simulink model "tutorial_picooz_simulation"  (R2024a)
settings: Solver=ode45  StartTime=0.0  StopTime=22  MaxStep=.002  RelTol=1e-3  EnableMultiTasking=on
undefined symbols (not defined in the file): DiscIntNeverNeededParam
libraries: simulink x2
settings Model: Creator=M91449  LastModifiedBy=Lubin Kerhuel
settings SolverCC: AlgebraicLoopSolver=TrustRegion
settings DataIOCC: ExternalInput=getinputstruct(op_trim1)  InitialState=getstatestruct(op_trim1)  SaveFormat=Array  SaveOutput=off  DSMLogging=off  SaveTime=off  ReturnWorkspaceOutputs=off
settings OptimizationCC: LifeSpan=inf
settings DebuggingCC: UnderspecifiedInitializationDetection=Classic  MergeDetectMultiDrivingBlocksExec=none  SolverPrmCheckMsg=warning  UnconnectedInputMsg=warning  UnconnectedOutputMsg=warning  UnconnectedLineMsg=warning  StateNameClashWarn=warning  SFUnexpectedBacktrackingDiag=warning  SFNoUnconditionalDefaultTransitionDiag=warning  SFExecutionAtInitializationDiag=none  ArithmeticOperatorsInVariantConditions=warning
settings HardwareCC: ProdBitPerPointer=32  ProdBitPerSizeT=32  ProdBitPerPtrDiffT=32  ProdLargestAtomicFloat=None  ProdIntDivRoundTo=Undefined  ProdEndianess=Unspecified  ProdWordSize=32  ProdHWDeviceType=32-bit Generic
settings ModelReferenceCC: PropagateSignalLabelsOutOfModel=off
settings SFSimCC: SimUseLocalCustomCode=off  CustomCodeUndefinedFunction=UseInterfaceOnly
settings RTWCC: RTWUseLocalCustomCode=off  GPUComputeCapability=3.5
settings CodeAppCC: StateflowObjectComments=on
settings GRTTargetCC: TargetLangStandard=C89/C90 (ANSI)
settings ConfigComp: CovMetricSettings=dw  CovSaveCumulativeToWorkspaceVar=on  CovSaveSingleToWorkspaceVar=on  CovExternalEMLEnable=off  CovSFcnEnable=off

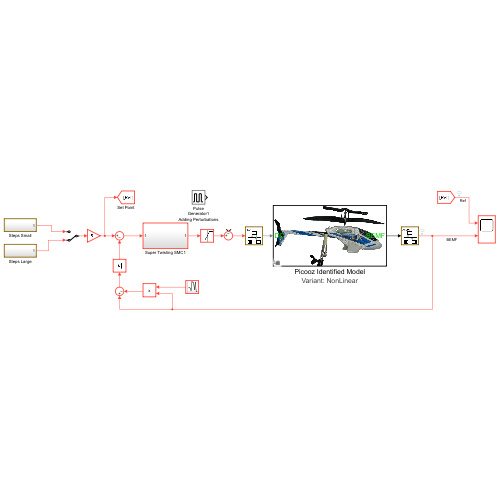
[thumbnail: Simulink's stored preview of the top-level diagram]
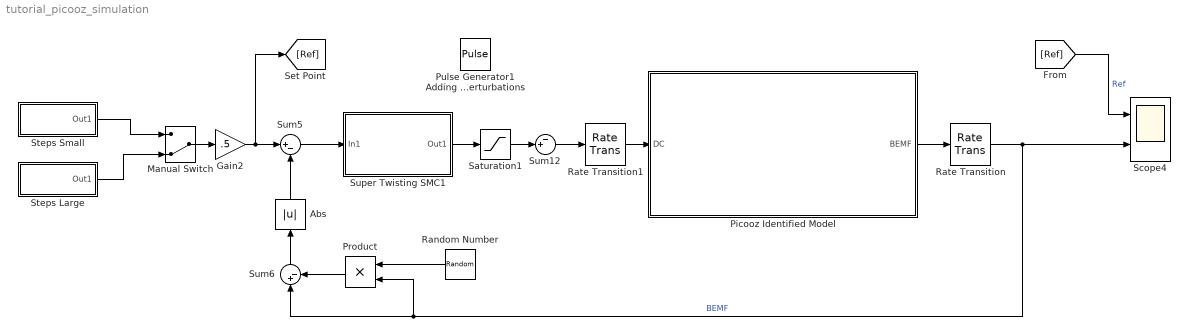
== system tutorial_picooz_simulation ==
  Abs : Abs  SaturateOnIntegerOverflow=off
  Gain2 : Gain  Gain=.5  OutDataTypeStr=double
  Manual Switch : ManualSwitch  CurrentSetting=0
  Picooz Identified Model : Subsystem  Variant=on  VariantControlMode=label  LabelModeActiveChoice=NonLinear
      settings: AttributesFormatString=Variant: %<ActiveVariant>
      mask Display:
      | color('green');
      | image('Picooz_01_Close.jpg');
      | port_label('input',1,'DC');
      | port_label('output',1,'BEMF');
      | %disp(get_param(gcb,'ActiveVariant'));
  Product : Product
  Pulse Generator1 Adding Perturbations : DiscretePulseGenerator  PulseType=Time based  Amplitude=.15  Period=2.3  PulseWidth=10
  Random Number : RandomNumber  Variance=.012^2*5  SampleTime=0.001
  Rate Transition : RateTransition  OutPortSampleTime=.001
  Rate Transition1 : RateTransition  OutPortSampleTime=0
  Saturation1 : Saturate  UpperLimit=.8  LowerLimit=0
  Scope4 : Scope  NumInputPorts=2
  Steps Large : Subsystem
  Steps Small : Subsystem
  Sum12 : Sum  Inputs=-+|  SampleTime=.001
  Sum5 : Sum  Inputs=|+-  SampleTime=.001
  Sum6 : Sum  Inputs=|+-
  Super Twisting SMC1 : Subsystem
  wires:
  Sum5/1 -> Super Twisting SMC1/1(In1)
  Picooz Identified Model/1(BEMF) -> Rate Transition/1
  Saturation1/1 -> Sum12/2
  Super Twisting SMC1/1(Out1) -> Saturation1/1
  Sum6/1 -> Abs/1
  Rate Transition1/1 -> Picooz Identified Model/1(DC)
  Sum12/1 -> Rate Transition1/1
  Steps Small/1(Out1) -> Manual Switch/1
  Manual Switch/1 -> Gain2/1
  Rate Transition/1 -> Scope4/2, Product/2, Sum6/1  "BEMF"
  Steps Large/1(Out1) -> Manual Switch/2
  Abs/1 -> Sum5/2
  Gain2/1 -> [Ref], Sum5/1
  [Ref] -> Scope4/1  "Ref"
  Random Number/1 -> Product/1
  Product/1 -> Sum6/2

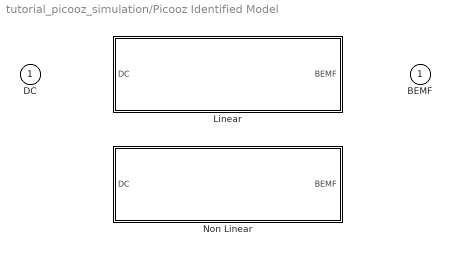
== system tutorial_picooz_simulation/Picooz Identified Model ==
  DC : Inport
  Linear : Subsystem  VariantControl=Linear
      mask Display:
      | disp('Linear Model');
      | port_label('input',1,'DC');
      | port_label('output',1,'BEMF');
  Non Linear : Subsystem  VariantControl=NonLinear
      mask Display:
      | disp('Non Linear Model')
      | color('green');
      | port_label('input',1,'DC');
      | port_label('output',1,'BEMF');
  BEMF : Outport

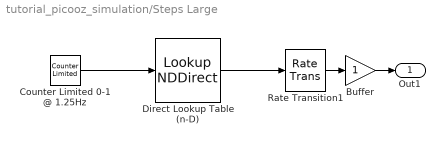
== system tutorial_picooz_simulation/Steps Large ==
  Buffer : Gain  OutDataTypeStr=Inherit: Same as input  ParamDataTypeStr=Inherit: Same as input
  Counter Limited 0-1 @ 1.25Hz : simulink/Sources/Counter Limited  uplimit=19  tsamp=1
  Direct Lookup Table (n-D) : LookupNDDirect  NumberOfTableDimensions=1  Table=[0 0 10 20 30 40 50 60 70 80 70 60 50 40 30 20 10 0 50 80] * 1 / 100  TableDataTypeStr=double
  Rate Transition1 : RateTransition  Integrity=off  Deterministic=off
  Out1 : Outport
  wires:
  Rate Transition1/1 -> Buffer/1
  Counter Limited 0-1 @ 1.25Hz/1 -> Direct Lookup Table (n-D)/1
  Direct Lookup Table (n-D)/1 -> Rate Transition1/1
  Buffer/1 -> Out1/1

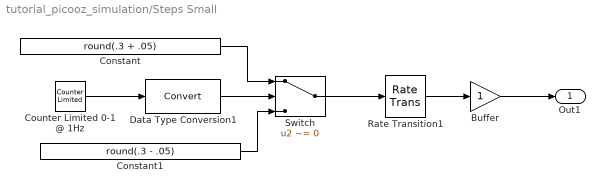
== system tutorial_picooz_simulation/Steps Small ==
  Buffer : Gain  OutDataTypeStr=Inherit: Same as input  ParamDataTypeStr=Inherit: Same as input
  Constant : Constant  Value=round(.3 + .05)  OutDataTypeStr=double
  Constant1 : Constant  Value=round(.3 - .05)  OutDataTypeStr=double
  Counter Limited 0-1 @ 1Hz : simulink/Sources/Counter Limited  uplimit=1  tsamp=1
  Data Type Conversion1 : DataTypeConversion  SaturateOnIntegerOverflow=off  RndMeth=Floor
  Rate Transition1 : RateTransition  Integrity=off  Deterministic=off
  Switch : Switch  Criteria=u2 ~= 0  SaturateOnIntegerOverflow=off  InputSameDT=off
  Out1 : Outport
  wires:
  Constant1/1 -> Switch/3
  Data Type Conversion1/1 -> Switch/2
  Switch/1 -> Rate Transition1/1
  Constant/1 -> Switch/1
  Counter Limited 0-1 @ 1Hz/1 -> Data Type Conversion1/1
  Rate Transition1/1 -> Buffer/1
  Buffer/1 -> Out1/1

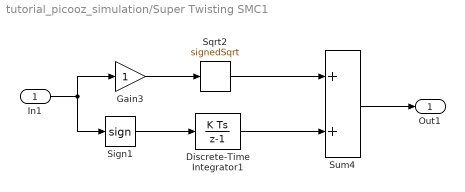
== system tutorial_picooz_simulation/Super Twisting SMC1 ==
  In1 : Inport
  Discrete-Time Integrator1 : DiscreteIntegrator  gainval=4  SampleTime=.001  LimitOutput=on  UpperSaturationLimit=1  LowerSaturationLimit=0  ICPrevOutput=DiscIntNeverNeededParam  ICPrevScaledInput=DiscIntNeverNeededParam
  Gain3 : Gain  OutDataTypeStr=double
  Sign1 : Signum
  Sqrt2 : Sqrt  Operator=signedSqrt
  Sum4 : Sum  SampleTime=.001
  Out1 : Outport
  wires:
  Sign1/1 -> Discrete-Time Integrator1/1
  Sum4/1 -> Out1/1
  In1/1 -> Gain3/1, Sign1/1
  Sqrt2/1 -> Sum4/1
  Discrete-Time Integrator1/1 -> Sum4/2
  Gain3/1 -> Sqrt2/1

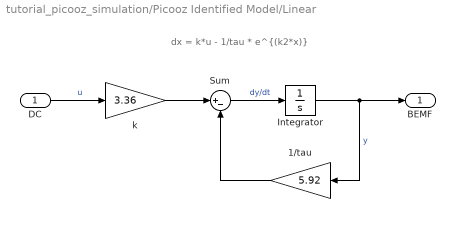
== system tutorial_picooz_simulation/Picooz Identified Model/Linear ==
  note: dx = k*u - 1/tau * e^{(k2*x)}
  DC : Inport
  1/tau : Gain  Gain=5.92
  Integrator : Integrator  LowerSaturationLimit=0
  Sum : Sum  Inputs=|+-
  k : Gain  Gain=3.36
  BEMF : Outport
  wires:
  Sum/1 -> Integrator/1  "dy/dt"
  1/tau/1 -> Sum/2
  k/1 -> Sum/1
  DC/1 -> k/1  "u"
  Integrator/1 -> BEMF/1, 1/tau/1  "y"

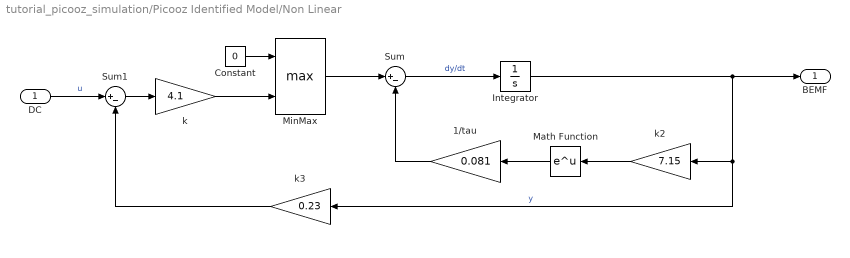
== system tutorial_picooz_simulation/Picooz Identified Model/Non Linear ==
  DC : Inport
  1/tau : Gain  Gain=0.081
  Constant : Constant  Value=0
  Integrator : Integrator  LimitOutput=on  LowerSaturationLimit=0
  Math Function : Math  SignedPower=on
  MinMax : MinMax  Function=max  Inputs=2  ZeroCross=off
  Sum : Sum  Inputs=|+-
  Sum1 : Sum  Inputs=|+-
  k : Gain  Gain=4.1
  k2 : Gain  Gain=7.15
  k3 : Gain  Gain=0.23
  BEMF : Outport
  wires:
  Math Function/1 -> 1/tau/1
  k2/1 -> Math Function/1
  Integrator/1 -> k2/1, k3/1, BEMF/1  "y"
  1/tau/1 -> Sum/2
  Sum/1 -> Integrator/1  "dy/dt"
  Constant/1 -> MinMax/1
  DC/1 -> Sum1/1  "u"
  Sum1/1 -> k/1
  k/1 -> MinMax/2
  MinMax/1 -> Sum/1
  k3/1 -> Sum1/2
